simulink model "hethongphanhABS"  (R2022b)
settings: Solver=VariableStepAuto  StartTime=0.0  StopTime=10.0  RelTol=1e-3
undefined symbols (not defined in the file): g, I, m, R, v0
settings Model: Creator=MyPC  LastModifiedBy=MyPC

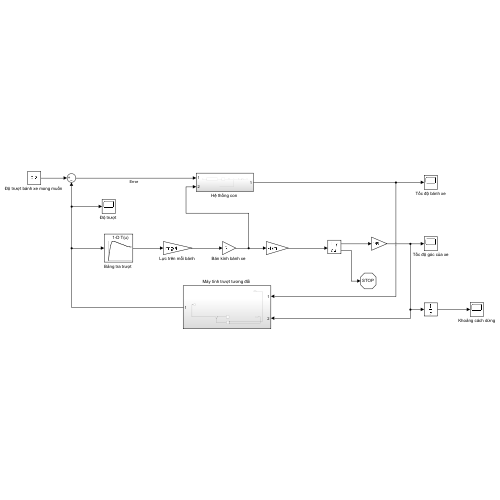
[thumbnail: Simulink's stored preview of the top-level diagram]
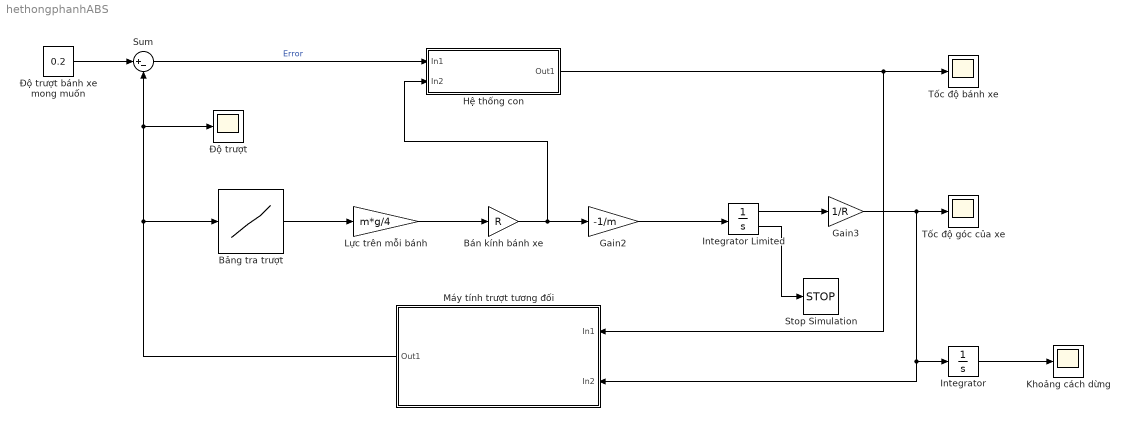
== system hethongphanhABS ==
  "Bán kính bánh xe " : Gain  Gain=R
  "Bảng tra trượt " : Lookup_n-D  NumberOfTableDimensions=1  LookupTableObject=''  BreakpointsForDimension1=[0,0.05,0.1,0.15,0.2,0.25,0.3,0.35,0.4,0.45,0.5,0.55,0.6,0.65,0.7,0.75,0.8,0.85,0.9,0.95,1]  BreakpointsForDimension1FirstPoint=10  BreakpointsForDimension2FirstPoint=10  BreakpointsForDimension1Spacing=12  BreakpointsForDimension2Spacing=12  Table=[0,0.4,0.8,0.97,1,0.98,0.96,0.94,0.92,0.9,0.88,0.855,0.83,0.81,0.79,0.77,0.75,0.73,0.72,0.71,0.7]  InternalRulePriority=Speed  RndMeth=Simplest
  Gain2 : Gain  Gain=-1/m
  Gain3 : Gain  Gain=1/R
  "Hệ thống con " : Subsystem
  Integrator : Integrator
  Integrator Limited : Integrator  InitialCondition=v0  LimitOutput=on  UpperSaturationLimit=1000  LowerSaturationLimit=0  ShowSaturationPort=on
  Khoảng cách dừng : Scope
  "Lực trên mỗi bánh " : Gain  Gain=m*g/4
  "Máy tính trượt tương đối " : Subsystem
  Stop Simulation : Stop
  Sum : Sum  Inputs=|+-
  Tốc độ bánh xe : Scope
  Tốc độ góc của xe : Scope
  "Độ trượt " : Scope
  "Độ trượt bánh xe mong muốn " : Constant  Value=0.2
  wires:
  "Độ trượt bánh xe mong muốn "/1 -> Sum/1
  Sum/1 -> "Hệ thống con "/1(In1)  "Error"
  "Bảng tra trượt "/1 -> "Lực trên mỗi bánh "/1
  "Lực trên mỗi bánh "/1 -> "Bán kính bánh xe "/1
  "Bán kính bánh xe "/1 -> "Hệ thống con "/2(In2), Gain2/1
  Gain2/1 -> Integrator Limited/1
  Integrator Limited/1 -> Gain3/1
  Integrator Limited/2 -> Stop Simulation/1
  "Hệ thống con "/1(Out1) -> Tốc độ bánh xe/1, "Máy tính trượt tương đối "/1(In1)
  Gain3/1 -> "Máy tính trượt tương đối "/2(In2), Integrator/1, Tốc độ góc của xe/1
  Integrator/1 -> Khoảng cách dừng/1
  "Máy tính trượt tương đối "/1(Out1) -> "Bảng tra trượt "/1, Sum/2, "Độ trượt "/1

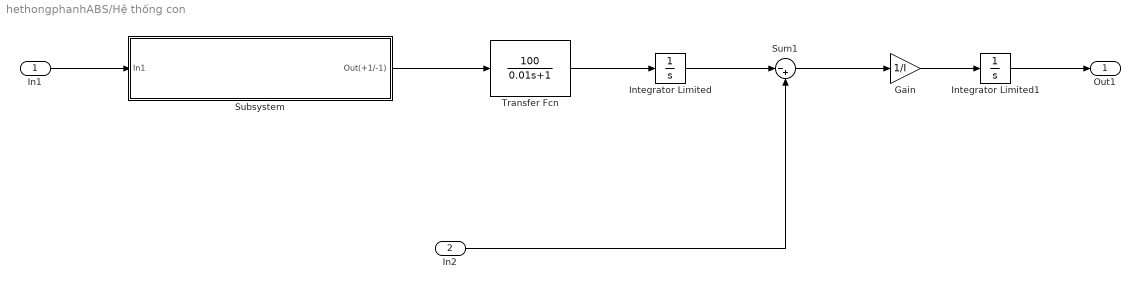
== system hethongphanhABS/Hệ thống con  ==
  In1 : Inport
  In2 : Inport  Port=2
  Gain : Gain  Gain=1/I
  Integrator Limited : Integrator  LimitOutput=on  UpperSaturationLimit=1000  LowerSaturationLimit=0
  Integrator Limited1 : Integrator  InitialCondition=v0/R  LimitOutput=on  UpperSaturationLimit=1000  LowerSaturationLimit=0
  Subsystem : Subsystem
  Sum1 : Sum  Inputs=|-+
  Transfer Fcn : TransferFcn  Numerator=[100]  Denominator=[0.01 1]
  Out1 : Outport
  wires:
  Integrator Limited/1 -> Sum1/1
  Integrator Limited1/1 -> Out1/1
  Transfer Fcn/1 -> Integrator Limited/1
  Sum1/1 -> Gain/1
  Gain/1 -> Integrator Limited1/1
  Subsystem/1(Out(+1/-1)) -> Transfer Fcn/1
  In2/1 -> Sum1/2
  In1/1 -> Subsystem/1(In1)

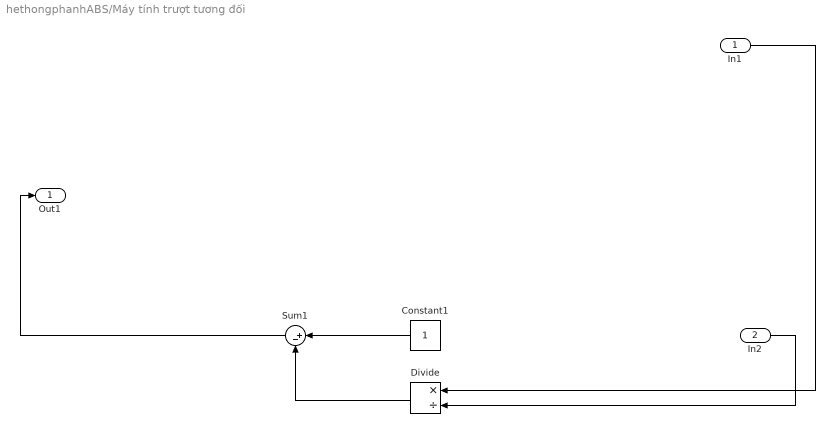
== system hethongphanhABS/Máy tính trượt tương đối  ==
  In1 : Inport
  In2 : Inport  Port=2
  Constant1 : Constant
  Divide : Product  Inputs=*/
  Sum1 : Sum  Inputs=|+-
  Out1 : Outport
  wires:
  Constant1/1 -> Sum1/1
  Divide/1 -> Sum1/2
  In2/1 -> Divide/2
  Sum1/1 -> Out1/1
  In1/1 -> Divide/1

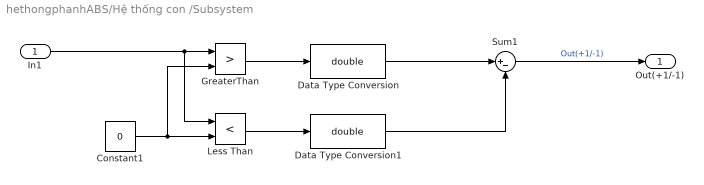
== system hethongphanhABS/Hệ thống con /Subsystem ==
  In1 : Inport
  Constant1 : Constant  Value=0
  Data Type Conversion : DataTypeConversion  OutDataTypeStr=double  SaturateOnIntegerOverflow=off
  Data Type Conversion1 : DataTypeConversion  OutDataTypeStr=double  SaturateOnIntegerOverflow=off
  GreaterThan : RelationalOperator  Operator=>  OutDataTypeStr=boolean  RndMeth=Simplest  InputSameDT=off
  Less Than : RelationalOperator  Operator=<  OutDataTypeStr=boolean  RndMeth=Simplest  InputSameDT=off
  Sum1 : Sum  Inputs=|+-
  Out(+1/-1) : Outport
  wires:
  GreaterThan/1 -> Data Type Conversion/1
  Data Type Conversion/1 -> Sum1/1
  Constant1/1 -> GreaterThan/2, Less Than/2
  In1/1 -> Less Than/1, GreaterThan/1
  Less Than/1 -> Data Type Conversion1/1
  Data Type Conversion1/1 -> Sum1/2
  Sum1/1 -> Out(+1/-1)/1  "Out(+1/-1)"
